simulink model "controller_arduino"  (R2024a)
settings: Solver=FixedStepAuto  StartTime=0.0  StopTime=10.0  FixedStep=1/10  RelTol=1e-3
libraries: arduinolib x9
settings Model: ExtModeTrigDuration=2  Creator=lucap  LastModifiedBy=lucap
settings SolverCC: AutoInsertRateTranBlk=on
settings OptimizationCC: EnhancedBackFolding=on  PassReuseOutputArgsAs=Individual arguments  ZeroExternalMemoryAtStartup=off  ZeroInternalMemoryAtStartup=off  MaxStackSize=64  OptimizeBlockOrder=speed  DifferentSizesBufferReuse=on  OptimizationCustomize=off  EfficientTunableParamExpr=on
settings DebuggingCC: ParameterTunabilityLossMsg=error
settings HardwareCC: ProdBitPerInt=16  ProdBitPerPointer=16  ProdBitPerSizeT=16  ProdBitPerPtrDiffT=16  ProdLargestAtomicFloat=None  ProdWordSize=8  ProdHWDeviceType=Atmel->AVR  UseEmbeddedCoderFeatures=off  UseSimulinkCoderFeatures=off
settings SFSimCC: MATLABDynamicMemAlloc=off
settings RTWCC: Description=Embedded Coder  SystemTargetFile=ert.tlc  HardwareBoard=Arduino Uno  TemplateMakefile=ert_default_tmf  Toolchain=Arduino AVR
settings CodeAppCC: ForceParamTrailComments=on  IgnoreCustomStorageClasses=off  OperatorAnnotations=on  SimulinkDataObjDesc=on  SFDataObjDesc=on  InsertBlockDesc=on
settings ERTTargetCC: SupportContinuousTime=on  SupportNonInlinedSFcns=on  SupportVariableSizeSignals=on  ExtModeTransport=3  ExtModeStaticAlloc=on  ExtModeAutomaticAllocSize=off  ExtModeStaticAllocSize=250  ExtModeMexFile=ext_xcp  ExtModeIntrfLevel=Level2 - Open

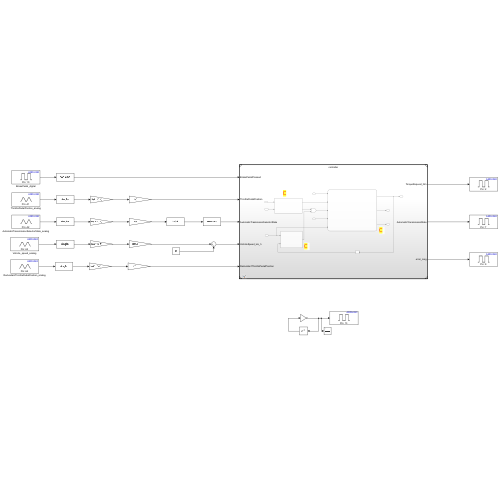
[thumbnail: Simulink's stored preview of the top-level diagram]
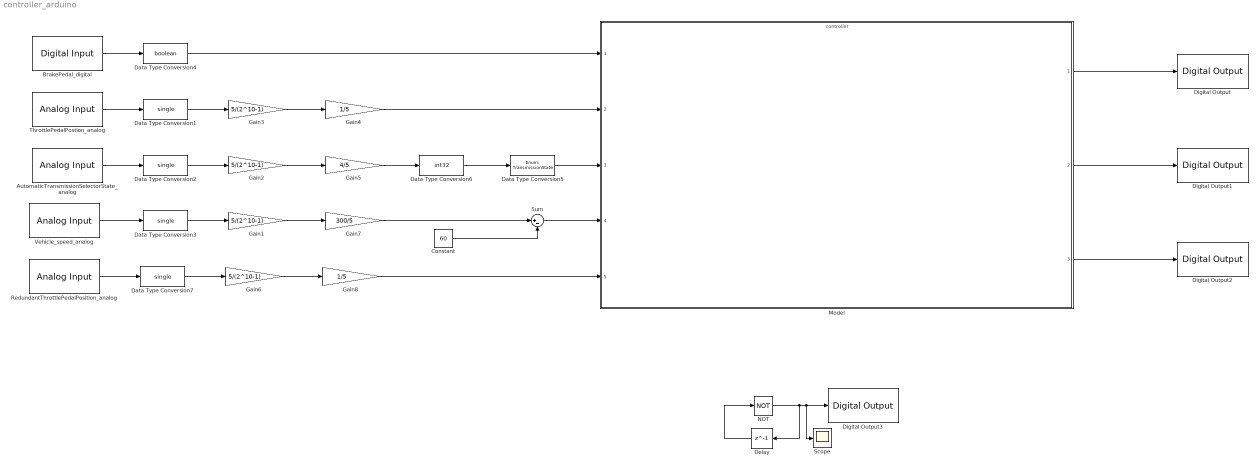
== system controller_arduino ==
  AutomaticTransmissionSelectorState_analog : arduinolib/Analog Input  pinNumber=2  ReadResultsOnly=off  ConversionTriggerSource=Software  ExternalTriggerType=uint32( 0 )  OutputDataType=uint16  EnableConversionCompleteNotify=off  EnableOuputStatus=off  SampleTime=-1  blockPlatform=arduino
  BrakePedal_digital : arduinolib/Digital Input  pinNumber=10  mode=Default  Direction=input  SampleTime=0.1  blockPlatform=arduino
  Constant : Constant  Value=60  OutDataTypeStr=single
  Data Type Conversion{1..3,7} (4 alike) : DataTypeConversion  OutDataTypeStr=single  SaturateOnIntegerOverflow=off  RndMeth=Floor
  Data Type Conversion4 : DataTypeConversion  OutDataTypeStr=boolean  SaturateOnIntegerOverflow=off  RndMeth=Floor  LockScale=on
  Data Type Conversion5 : DataTypeConversion  OutDataTypeStr=Enum: TransmissionState  SaturateOnIntegerOverflow=off  RndMeth=Floor  LockScale=on
  Data Type Conversion6 : DataTypeConversion  OutDataTypeStr=int32  SaturateOnIntegerOverflow=off  RndMeth=Floor
  Delay : Delay  DelayLength=1  SampleTime=0.5
  Digital Output : arduinolib/Digital Output  pinNumber=2  Direction=output  blockPlatform=arduino
  Digital Output1 : arduinolib/Digital Output  pinNumber=7  Direction=output  blockPlatform=arduino
  Digital Output2 : arduinolib/Digital Output  pinNumber=9  Direction=output  blockPlatform=arduino
  Digital Output3 : arduinolib/Digital Output  pinNumber=13  Direction=output  blockPlatform=arduino
  Gain{1..3,6} (4 alike) : Gain  Gain=5/(2^10-1)
  Gain4 : Gain  Gain=1/5
  Gain5 : Gain  Gain=4/5
  Gain7 : Gain  Gain=300/5
  Gain8 : Gain  Gain=1/5
  Model : ModelReference  ModelNameDialog=controller.slx  SimulationMode=Normal  ModelReferenceVersion=6.24
  NOT : Logic  Operator=NOT  IconShape=distinctive  AllPortsSameDT=off  OutDataTypeStr=boolean
  RedundantThrottlePedalPosition_analog : arduinolib/Analog Input  pinNumber=4  ReadResultsOnly=off  ConversionTriggerSource=Software  ExternalTriggerType=uint32( 0 )  OutputDataType=uint16  EnableConversionCompleteNotify=off  EnableOuputStatus=off  SampleTime=-1  blockPlatform=arduino
  Scope : Scope
  Sum : Sum  Inputs=|+-
  ThrottlePedalPostion_analog : arduinolib/Analog Input  pinNumber=1  ReadResultsOnly=off  ConversionTriggerSource=Software  ExternalTriggerType=uint32( 0 )  OutputDataType=uint16  EnableConversionCompleteNotify=off  EnableOuputStatus=off  SampleTime=-1  blockPlatform=arduino
  Vehicle_speed_analog : arduinolib/Analog Input  pinNumber=3  ReadResultsOnly=off  ConversionTriggerSource=Software  ExternalTriggerType=uint32( 0 )  OutputDataType=uint16  EnableConversionCompleteNotify=off  EnableOuputStatus=off  SampleTime=-1  blockPlatform=arduino
  wires:
  Delay/1 -> NOT/1
  NOT/1 -> Delay/1, Scope/1, Digital Output3/1
  Model/2 -> Digital Output1/1
  Model/1 -> Digital Output/1
  Vehicle_speed_analog/1 -> Data Type Conversion3/1
  ThrottlePedalPostion_analog/1 -> Data Type Conversion1/1
  Data Type Conversion3/1 -> Gain1/1
  Data Type Conversion1/1 -> Gain3/1
  Gain3/1 -> Gain4/1
  Gain1/1 -> Gain7/1
  Gain7/1 -> Sum/1
  Sum/1 -> Model/4
  Constant/1 -> Sum/2
  BrakePedal_digital/1 -> Data Type Conversion4/1
  Data Type Conversion5/1 -> Model/3
  Gain2/1 -> Gain5/1
  Gain5/1 -> Data Type Conversion6/1
  AutomaticTransmissionSelectorState_analog/1 -> Data Type Conversion2/1
  Data Type Conversion2/1 -> Gain2/1
  Data Type Conversion6/1 -> Data Type Conversion5/1
  Gain4/1 -> Model/2
  Data Type Conversion4/1 -> Model/1
  RedundantThrottlePedalPosition_analog/1 -> Data Type Conversion7/1
  Data Type Conversion7/1 -> Gain6/1
  Gain6/1 -> Gain8/1
  Gain8/1 -> Model/5
  Model/3 -> Digital Output2/1
